simulink model "MPS_device_passive"  (R2018b)
settings: Solver=ode4  StartTime=0  StopTime=700  FixedStep=0.02  MaxStep=0.02  RelTol=1e-3  EnableMultiTasking=on
InitFcn:
  | %SSModel_calc
undefined symbols (not defined in the file): body, CentralPTOPreload, constraint, L, ML1Preload, ML2Preload, ML3Preload, ML4Preload, ML5Preload, ML6Preload, ML7Preload, ML8Preload, mrelative, pto, PTOrotation, SidePTO1Preload, SidePTO2Preload, SidePTO3Preload, SidePTO4Preload, simu, waves, X, Y, Z
libraries: nesl_utility x580, sm_lib x317, vrlib x72, WECSim_Lib x36
(part 26 of 27)

== matlab function MPS_device_passive/Control/Inverse Kinematic Jacobian - dynamic Go from 4 line forces to 6 Cartesian forces ==
  data: u input; y output
%Transform velocity or force from line space to cartesian space
%(underdetermined)

function y = dynamic_L(u)

rho_sea=1000;
g=9.81;
% Float
depth = 2;                  % Depth to top of float
Des = 12;                   % Outer diameter of float shell [m]
R = Des/2;                  % Outer radius of float shell [m]
CylLength = 4.75;           % Length of cylinder between hemispheres [m]
reldenfloat = 0.8;          % Density of float reative to sea water [-]
rho_steel = 7850;           % Density of steel [kg/m^3]
alphaDeg = 45;               % deg xz-plane (zero if att point is on horizontal central line, 90 if on bottom og float)
betaDeg = 0;               % deg xy-plane (zero if x value of att point is max (corner of cylinder) 90 y is max (peak of hemisphere))
FloatCd = 0.5;
FloatCdVector = [FloatCd 100 FloatCd 200*FloatCd 0 200*FloatCd];% Drag coefficients in 6 degrees of freedom, 4 and 6 picked at random to reduce yaw movement

% Reactor
ReactorD = 4.3;
ReactorCylLength = 35.7;                        % Only cylinder (excluding the two hemispheres)
ReactorWidth = 30;                              % From centre of tube to centre of tube
NetBuoyReactor = 101.9*10^3;                    % Net buoyancy of reactor [f kg] (Positive is buoyant)
ReactorDepth = 25.85;                           % Distance from mean sea surface to top of reactor (positive nr)
SeaDepth = 75;                                  % Distance from mean sea surface to seabed (positive nr)
ReactorCd = 0.5;
ReactorCdVector = [ReactorCd 100 ReactorCd 200*ReactorCd 200*ReactorCd 200*ReactorCd];   % Drag coefficients in 6 degrees of freedom, 4 and 6 picked at random to reduce yaw movement

%% Coordinates  (m, m, m)
% Tether line attachemnt point on float in global frame
%Transform to Float local frame - subtract float radius from z co-ord
%(Global frame at sea level)
F1 = [u(1) u(2) u(3)+8];
F2 = [u(4) u(5) u(6)+8];     % Corner tether
F3 = [u(7) u(8) u(9)+8];    % Corner tether
F4 = [u(10) u(11) u(12)+8];     % Corner tether

% Tether line attachemnt point on reactor in global frame
T1 = [ReactorCylLength/2 ReactorWidth/2 -ReactorDepth+depth+R];      % Corner tether transformed to relative to float COG
T2 = [T1(1) -T1(2) T1(3)];               % Corner tether
T3 = [-T1(1) -T1(2) T1(3)];              % Corner tether
T4 = [-T1(1) T1(2) T1(3)];               % Corner tether

%Vectors to float thether attachment points relative to float COG
N_01=[0 F1(3) -F1(2);-F1(3) 0 F1(1);F1(2) -F1(1) 0];
N_02=[0 F2(3) -F2(2);-F2(3) 0 F2(1);F2(2) -F2(1) 0];
N_03=[0 F3(3) -F3(2);-F3(3) 0 F3(1);F3(2) -F3(1) 0];
N_04=[0 F4(3) -F4(2);-F4(3) 0 F4(1);F4(2) -F4(1) 0];

%Vectors along PTO tethers
S1=F1-T1;
S2=F2-T2;
S3=F3-T3;
S4=F4-T4;

S_01=[0 S1(3) -S1(2);-S1(3) 0 S1(1);S1(2) -S1(1) 0];
S_02=[0 S2(3) -S2(2);-S2(3) 0 S2(1);S2(2) -S2(1) 0];
S_03=[0 S3(3) -S3(2);-S3(3) 0 S3(1);S3(2) -S3(1) 0];
S_04=[0 S4(3) -S4(2);-S4(3) 0 S4(1);S4(2) -S4(1) 0];

%Unit vectors along PTO tethers
e_s1=S1./norm(S1);
e_s2=S2./norm(S2);
e_s3=S3./norm(S3);
e_s4=S4./norm(S4);


%%%%Kt for non colinear lines
G_01 = -[eye(3);N_01']*e_s1';
G_02 = -[eye(3);N_02']*e_s2';
G_03 = -[eye(3);N_03']*e_s3';
G_04 = -[eye(3);N_04']*e_s4';

%Inverse kinematic Jacobian
L = -[G_01 G_02 G_03 G_04]';
y = L';

== matlab function MPS_device_passive/PTO P1F1/VisuP1F2/Hydrodynamic Body/Nonlinear Wave Elevation/Linear or Instantaneous Free Surface/Instantaneous Water Free Surface  /Instantaneous FS ==
  data: x input; center input; f output; cg input; AH input; w input; dw input; k input; typeNum input; t input; rampT input; phaseRand input; waveDir input; dt input; dtFe input
function f  = waveElevation(x,center,cg,AH,w,dw,k,typeNum,t,rampT,phaseRand,waveDir, dt, dtFe)
    % Function to calculate the wave elevation at the ceontroids of triangulated surface
    % NOTE: This function assumes that the STL file is imported with its CG at 0,0,0
    persistent oldElev
    if isempty(oldElev)
        f = calc_elev(x,center,cg,AH,w,dw,k,typeNum,t,rampT,phaseRand, waveDir);
        oldElev = f;
    else
        if mod(t, dtFe) < dt/2
            f = calc_elev(x,center,cg,AH,w,dw,k,typeNum,t,rampT,phaseRand, waveDir);
            oldElev = f;
        else
            f = oldElev;
        end
    end
end

function f = calc_elev(x,center,cg,AH,w,dw,k,typeNum,t,rampT,phaseRand,waveDir)
    % Function to rotate and translate body and call wave elevation function at new locations 
    
    % Compute new tri center coords after cog rotation and translation
    center = rotateXYZ(center,[1 0 0],x(4));
    center = rotateXYZ(center,[0 1 0],x(5));
    center = rotateXYZ(center,[0 0 1],x(6));
    center = offsetXYZ(center,x);
    center = offsetXYZ(center,cg);
    % Calculate the free surface
    f=waveElev(center,AH,w,dw,t,k,rampT,phaseRand,typeNum,waveDir);
end

function verts = offsetXYZ(verts,x)
    % Function to move the position vertices
    verts(:,1) = verts(:,1) + x(1);
    verts(:,2) = verts(:,2) + x(2);
    verts(:,3) = verts(:,3) + x(3);
end

function xn = rotateXYZ(x,ax,t)
	% Function to rotate a point about an arbitrary axis
	% x: 3-component coordinates
	% ax: axis about which to rotate (must be a vector length 1)
	% t: rotation angle
	% xn: new coordinates after rotation
	rotMat = zeros(3);
	rotMat(1,1) = ax(1)*ax(1)*(1-cos(t))    + cos(t);
	rotMat(1,2) = ax(2)*ax(1)*(1-cos(t))    + ax(3)*sin(t);
	rotMat(1,3) = ax(3)*ax(1)*(1-cos(t))    - ax(2)*sin(t);
	rotMat(2,1) = ax(1)*ax(2)*(1-cos(t))    - ax(3)*sin(t);
	rotMat(2,2) = ax(2)*ax(2)*(1-cos(t))    + cos(t);
	rotMat(2,3) = ax(3)*ax(2)*(1-cos(t))    + ax(1)*sin(t);
	rotMat(3,1) = ax(1)*ax(3)*(1-cos(t))    + ax(2)*sin(t);
	rotMat(3,2) = ax(2)*ax(3)*(1-cos(t))    - ax(1)*sin(t);
	rotMat(3,3) = ax(3)*ax(3)*(1-cos(t))    + cos(t);
	xn = x*rotMat;
end

function f=waveElev(center,AH,w,dw,t,k,rampT,phaseRand,typeNum,waveDir)
    % Function to calculate the wave elevation at an array of points
    f = zeros(length(center(:,3)),1);
    cx = center(:,1);
    cy = center(:,2);
    X = cx*cos(waveDir*pi/180) + cy*sin(waveDir*pi/180);
    if typeNum <10
    elseif typeNum <20
        f = AH(1).*cos(k(1).*X-w(1)*t);
    elseif typeNum <30
        tmp=sqrt(AH.*dw);
        tmp1 = ones(1,length(center(:,1)));
        tmp2 = (w.*t+phaseRand)*tmp1;
        tmp3 = cos(k*X'- tmp2);
        f(:,1) = tmp3'*tmp;
    end
    if t<=rampT
        rampF = (1+cos(pi+pi*t/rampT))/2;
        f = f.*rampF;
    end
end

== matlab function MPS_device_passive/PTO P1F1/VisuP1F2/Hydrodynamic Body/Structure/Motion Sensor/Angle ==
  data: Q input; E output
function E  = EulerAngle(Q)
% Euler Angle Type II or Tait-Bryan Angle for sequence 321 or zyx (Nautical or Cardan angles).
% Yaw [-180,180], followed by pitch [-90,90], followed by roll [-180,180]
E = zeros(3,1);
E(1) = atan2((2*(Q(1)*Q(2)+Q(3)*Q(4))),(1-2*(Q(2)^2+Q(3)^2)));
E(2) = asin(2*(Q(1)*Q(3)-Q(4)*Q(2)));
E(3) = atan2((2*(Q(1)*Q(4)+Q(2)*Q(3))),(1-2*(Q(3)^2+Q(4)^2)));

== matlab function MPS_device_passive/PTO P1F1/VisuP1F2/Hydrodynamic Body/Wave Diffraction and Excitation Force Calculation/Linear Wave Excitation Force Variant Subsystem/Irregular Wave Excitation Force/MATLAB Function ==
  data: A input; Fext output; w input; fExtRE input; fExtIM input; phaseRand input; dw input; time input
function Fext = fcn(A,w,fExtRE,fExtIM,phaseRand,dw,time)
%#codegen

persistent A1 B1 B11 C1 D1 D11 E1 E11

A1=bsxfun(@plus,w*time,pi/2);
B1= sin(bsxfun(@plus,A1,phaseRand));
B11 = sin(bsxfun(@plus,w*time,phaseRand));
C1 = sqrt(bsxfun(@times,A,dw));
D1 =bsxfun(@times,fExtRE,C1);
D11 = bsxfun(@times,fExtIM,C1);
E1 = bsxfun(@times,B1,D1);
E11 = bsxfun(@times,B11,D11);

Fext = sum(bsxfun(@minus,E1,E11));

== matlab function MPS_device_passive/PTO P1F1/VisuP1F2/Hydrodynamic Body/Wave Diffraction and Excitation Force Calculation/Nonlinear FK Force Variant Subsystem/With Nonlinear FroudeKrylov Force/Diffraction and Excitation Forces ==
  data: x input; elv input; center input; f output; tnorm input; area input; rho input; g input; cg input; AH input; w input; dw input; wDepth input; deepWaterWave input; k input; typeNum input; t input; phaseRand input; wp output; wpMeanFS output; dt input; dtFe input
function [f, wp, wpMeanFS]  = nonFKForce(x,elv,center,tnorm,area,rho,g,cg,AH,w,dw,wDepth,deepWaterWave,k,typeNum,t,phaseRand, dt, dtFe)
    % Function to calculate wave exitation force and moment on a triangulated surface
    % NOTE: This function assumes that the STL file is imported with its CG at 0,0,0
    
    % Logic to calculate nonFKForce at reduced sample time
    persistent oldForce
    persistent oldWp
    persistent oldWpMeanFs
    
    if isempty(oldForce)
        [f, wp, wpMeanFS] = calc_force(x,elv,center,tnorm,area,rho,g,cg,AH,w,dw,wDepth,deepWaterWave,k,typeNum,t,phaseRand);
        oldForce = f;
        oldWp = wp;
        oldWpMeanFs = wpMeanFS;
    else
        if mod(t, dtFe) < dt/2
            [f, wp, wpMeanFS] = calc_force(x,elv,center,tnorm,area,rho,g,cg,AH,w,dw,wDepth,deepWaterWave,k,typeNum,t,phaseRand);
            oldForce = f;
            oldWp = wp;
            oldWpMeanFs = wpMeanFS;
        else
            f = oldForce;
            wp = oldWp;
            wpMeanFS = oldWpMeanFs;
        end
    end
end

function [f, wp, wpMeanFS]  = calc_force(x,elv,center,tnorm,area,rho,g,cg,AH,w,dw,wDepth,deepWaterWave,k,typeNum,t,phaseRand)
    % Function to apply translation and rotation, and calculate forces.
    
    % Compute new tri coords after cog rotation and translation
    centerMeanFS = offsetXYZ(center,cg);
    avMeanFS     = tnorm .* [area area area];
    
    % Compute new tri coords after cog rotation and translation
    center = rotateXYZ(center,[1 0 0],x(4));
    center = rotateXYZ(center,[0 1 0],x(5));
    center = rotateXYZ(center,[0 0 1],x(6));
    center = offsetXYZ(center,x);
    center = offsetXYZ(center,cg);
    % Compute new normal vectors coords after cog rotation and translation
    tnorm = rotateXYZ(tnorm,[1 0 0],x(4));
    tnorm = rotateXYZ(tnorm,[0 1 0],x(5));
    tnorm = rotateXYZ(tnorm,[0 0 1],x(6));
    
    % Copute area vectors
    av = tnorm .* [area area area];
    
    % Calculate the free surface
    wpMeanFS=pDis(centerMeanFS,       0,AH,w,dw,wDepth,deepWaterWave,t,k,phaseRand,typeNum,rho,g);
    wp      =pDis(center      ,     elv,AH,w,dw,wDepth,deepWaterWave,t,k,phaseRand,typeNum,rho,g);
    
    % Calculate forces
    f_linear   =FK(centerMeanFS,       cg,avMeanFS,wpMeanFS);
    f_nonLinear=FK(center      ,x(1:3)+cg,av      ,wp      ); 
    f = f_nonLinear-f_linear;
end

function verts = offsetXYZ(verts,x)
    % Function to move the position vertices
    verts(:,1) = verts(:,1) + x(1);
    verts(:,2) = verts(:,2) + x(2);
    verts(:,3) = verts(:,3) + x(3);
end

function xn = rotateXYZ(x,ax,t)
	% Function to rotate a point about an arbitrary axis
	% x: 3-componenet coordinates
	% ax: axis about which to rotate (must be a vector length 1)
	% t: rotation angle
	% xn: new coordinates after rotation
	rotMat = zeros(3);
	rotMat(1,1) = ax(1)*ax(1)*(1-cos(t))    + cos(t);
	rotMat(1,2) = ax(2)*ax(1)*(1-cos(t))    + ax(3)*sin(t);
	rotMat(1,3) = ax(3)*ax(1)*(1-cos(t))    - ax(2)*sin(t);
	rotMat(2,1) = ax(1)*ax(2)*(1-cos(t))    - ax(3)*sin(t);
	rotMat(2,2) = ax(2)*ax(2)*(1-cos(t))    + cos(t);
	rotMat(2,3) = ax(3)*ax(2)*(1-cos(t))    + ax(1)*sin(t);
	rotMat(3,1) = ax(1)*ax(3)*(1-cos(t))    + ax(2)*sin(t);
	rotMat(3,2) = ax(2)*ax(3)*(1-cos(t))    - ax(1)*sin(t);
	rotMat(3,3) = ax(3)*ax(3)*(1-cos(t))    + cos(t);
	xn = x*rotMat;
end

function f=pDis(center,elv,AH,w,dw,wDepth,deepWaterWave,t,k,phaseRand,typeNum,rho,g)
    % Function to calculate pressure distribution
    f = zeros(length(center(:,3)),1);
    z=zeros(length(center(:,1)),1);
    if typeNum <10
    elseif typeNum <20
        f = rho.*g.*AH(1).*cos(k(1).*center(:,1)-w(1)*t);
        if deepWaterWave == 0
            z=(center(:,3)-elv).*wDepth./(wDepth+elv);
            f = f.*(cosh(k(1).*(z+wDepth))./cosh(k(1)*wDepth));
        else
            z=(center(:,3)-elv);
            f = f.*exp(k(1).*z);
        end
    elseif typeNum <30
        for i=1:length(AH)
            if deepWaterWave == 0 && wDepth <= 0.5*pi/k(i)
                z=(center(:,3)-elv).*wDepth./(wDepth+elv);
                f_tmp = rho.*g.*sqrt(AH(i)*dw).*cos(k(i).*center(:,1)-w(i)*t-phaseRand(i));
                f = f + f_tmp.*(cosh(k(i).*(z+wDepth))./cosh(k(i).*wDepth));
            else
                z=(center(:,3)-elv);
                f_tmp = rho.*g.*sqrt(AH(i)*dw).*cos(k(i).*center(:,1)-w(i)*t-phaseRand(i));
                f = f + f_tmp.*exp(k(i).*z);
            end
        end
    end
    f(z>0)=0;
end

function f = FK(center,instcg,av,wp)
    % Function to calculate the force and moment about the cog due to Froude-Krylov pressure
    f = zeros(6,1);
    
    % Calculate the hydrostatic pressure at each triangle center
    pressureVect = [wp wp wp].*-av;
    
    % Compute force about cog
    f(1:3) = sum(pressureVect);
    
    % Compute moment about cog
    tmp1 = ones(length(center(:,1)),1);
    tmp2 = tmp1*instcg';
    center2cgVec = center-tmp2;
    
    f(4:6)= sum(cross(center2cgVec,pressureVect));
end

== matlab function MPS_device_passive/PTO P1F1/VisuP1F2/Hydrodynamic Body/Wave Radiation Forces Calculation/SS CI and Constant-Damping-CoeVariant Subsystem/Convolution Integral Calculation/Fluid Memory ==
  data: lenJ input; v input; F_FM output; IRKB input; CTTime input; clockTime input
function F_FM = ConvolutionIntegral(lenJ,v,IRKB,CTTime,clockTime)
% Function to calculate convolution integral
interp_factor = 1;
%define persistent variables
persistent velocity;
persistent oldTime;
persistent oldF_FM;
persistent IRKB_interp;

dt = CTTime(2)-CTTime(1);
len = length(CTTime);
lenJ=length(lenJ);

%update velocity
if isempty(velocity)
    velocity = zeros(lenJ,len);
    oldTime = 0;
    F_FM    = zeros(6,1);
    oldF_FM = zeros(6,1);
    IRKB_reordered = permute(IRKB,[3 1 2]);
    IRKB_interp    = IRKB_reordered(:,1:interp_factor:end, :);
else
    if abs(clockTime-oldTime-dt)<0.00000001
        velocity      = circshift(velocity, 1, 2);
        velocity(:,1) = v(:);
        %integrate       
        time_series = bsxfun(@times, IRKB_interp, velocity);
        F_FM =squeeze(trapz(CTTime,sum(time_series, 1)));
         oldF_FM = F_FM;
         oldTime = clockTime;
    else
        F_FM = oldF_FM;
    end
end

end

== matlab function MPS_device_passive/PTO P1F1/VisuP1F2/Non-Hydro Body/Structure/Motion Sensor/Angle ==
  data: Q input; E output
function E  = EulerAngle(Q)
% Euler Angle Type II or Tait-Bryan Angle for sequence 321 or zyx (Nautical or Cardan angles).
% Yaw [-180,180], followed by pitch [-90,90], followed by roll [-180,180]
E = zeros(3,1);
E(1) = atan2( (2*(Q(1)*Q(2)+Q(3)*Q(4))), (1-2* (Q(2)^2+Q(3)^2) ) );
E(2) = asin( 2* (Q(1)*Q(3) - Q(4)*Q(2)));
E(3) = atan2( (2*(Q(1)*Q(4)+Q(2)*Q(3))), (1-2* (Q(3)^2+Q(4)^2) ) );

== matlab function MPS_device_passive/PTO P2F2/VisuP2F3/Hydrodynamic Body/Hydrostatic Restoring Force Calculation/Linear and Nonlinear Restoring Force Variant Subsystem/Nonlinear Hydrostatic Restoring Force/Diffarction and Excitation Forces1 ==
  data: x input; elv input; center input; f output; tnorm input; area input; rho input; g input; cg input; p output; dt input; dtFe input; t input
function [f,p]  = nonLinearBuoyancy(x,elv,center,tnorm,area,rho,g,cg,dt,dtFe,t)
% Function to calculate buoyancy force and moment on a triangulated surface
% NOTE: This function assumes that the STL file is imported with its CG at 0,0,0
persistent oldF 
persistent oldP

if isempty(oldF)
    [f,p] = calc_buoyancy(x,elv,center,tnorm,area,rho,g,cg);
    oldF  = f;
    oldP  = p;
else
    if mod(t, dtFe) < dt/2
        [f,p] = calc_buoyancy(x,elv,center,tnorm,area,rho,g,cg);
        oldF  = f;
        oldP  = p;
    else
        f  = oldF;
        p  = oldP;
    end
end
end


function [f,p] = calc_buoyancy(x,elv,center,tnorm,area,rho,g,cg)
% Function to apply translation and rotation and calculate forces

% Compute new tri coords after cog rotation and translation
center = rotateXYZ(center,[1 0 0],x(4));
center = rotateXYZ(center,[0 1 0],x(5));
center = rotateXYZ(center,[0 0 1],x(6));
center = offsetXYZ(center,x);
center = offsetXYZ(center,cg);
% Compute new normal vectors coords after cog rotation
tnorm = rotateXYZ(tnorm,[1 0 0],x(4));
tnorm = rotateXYZ(tnorm,[0 1 0],x(5));
tnorm = rotateXYZ(tnorm,[0 0 1],x(6));

% Calculate the hydrostatic forces
av = tnorm .* [area area area];
[f,p]=fHydrostatic(center,elv,x(1:3)+cg,av,rho,g); 
end

function verts = offsetXYZ(verts,x)
% Function to move the position vertices
verts(:,1) = verts(:,1) + x(1);
verts(:,2) = verts(:,2) + x(2);
verts(:,3) = verts(:,3) + x(3);
end

function xn = rotateXYZ(x,ax,t)
	% Function to rotate a point about an arbitrary axis
	% x: 3-componenet coordiantes
	% ax: axis about which to rotate (must be a vector length 1)
	% t: rotation angle
	% xn: new coordinates after rotation
	rotMat = zeros(3);
	rotMat(1,1) = ax(1)*ax(1)*(1-cos(t))    + cos(t);
	rotMat(1,2) = ax(2)*ax(1)*(1-cos(t))    + ax(3)*sin(t);
	rotMat(1,3) = ax(3)*ax(1)*(1-cos(t))    - ax(2)*sin(t);
	rotMat(2,1) = ax(1)*ax(2)*(1-cos(t))    - ax(3)*sin(t);
	rotMat(2,2) = ax(2)*ax(2)*(1-cos(t))    + cos(t);
	rotMat(2,3) = ax(3)*ax(2)*(1-cos(t))    + ax(1)*sin(t);
	rotMat(3,1) = ax(1)*ax(3)*(1-cos(t))    + ax(2)*sin(t);
	rotMat(3,2) = ax(2)*ax(3)*(1-cos(t))    - ax(1)*sin(t);
	rotMat(3,3) = ax(3)*ax(3)*(1-cos(t))    + cos(t);
	xn = x*rotMat;
end

function [f,p] = fHydrostatic(center,elv,instcg,av,rho,g)
% Function to calculate the force and moment about the cog due to hydrostatic pressure
f = zeros(6,1);

% Zeor out regions above the mean free surface
z=center(:,3); z((z-elv)>0)=0;

% Calculate the hydrostatic pressure at each triangle center
pressureVect = rho*g.*[-z -z -z].*-av;
p = rho*g.*-z;
% Compute force about cog
f(1:3) = sum(pressureVect);

tmp1 = ones(length(center(:,1)),1);
tmp2 = tmp1*instcg';
center2cgVec = center-tmp2;

f(4:6)= sum(cross(center2cgVec,pressureVect));
end

== matlab function MPS_device_passive/PTO P2F2/VisuP2F3/Hydrodynamic Body/Morrison Element and ViscousDampingForceCalculation/Morrison Element Variant Subsystem/Morrison Element On/Irregular Wave Morison Force/MorrisonElements/MorisonElementIrregular/MATLAB Function ==
  data: u output; v output; disp input size=[1 3]; waveNumber input; waveFreq input; waveAmp input; randPhase input; time input; rampT input size=[1 1]; waveDir input size=[1 1]; waterDepth input size=[1 1]; g input size=[1 1]; w output; xa output; ya output; za output
function [u,v,w,xa,ya,za] = calc_orbital_vel(disp, waveNumber, waveFreq, waveAmp, randPhase, time, rampT, waveDir, waterDepth, g)
%#codegen

[u,v,w,xa,ya,za] = orbital_velocity(disp, waveNumber, waveFreq, waveAmp, randPhase, time, rampT, waveDir, waterDepth, g);

== matlab function MPS_device_passive/PTO P2F2/VisuP2F3/Hydrodynamic Body/Morrison Element and ViscousDampingForceCalculation/Morrison Element Variant Subsystem/Morrison Element On/Regular Wave Morison Force/MorrisonElements/OrbitalVelocity/MATLAB Function ==
  data: u output; v output; disp input size=[1 3]; waveNumber input size=[1 1]; waveFreq input size=[1 1]; waveAmp input size=[1 1]; randPhase input; time input; rampT input size=[1 1]; waveDir input size=[1 1]; waterDepth input size=[1 1]; g input size=[1 1]; w output; xa output; ya output; za output
function [u,v,w,xa,ya,za] = calc_orbital_vel(disp, waveNumber, waveFreq, waveAmp, randPhase, time, rampT, waveDir, waterDepth, g)
%#codegen

[u,v,w,xa,ya,za] = orbital_velocity(disp, waveNumber, waveFreq, waveAmp, randPhase, time, rampT, waveDir, waterDepth, g);

== matlab function MPS_device_passive/PTO P2F2/VisuP2F3/Hydrodynamic Body/Nonlinear Wave Elevation/Linear or Instantaneous Free Surface/Instantaneous Water Free Surface  /Instantaneous FS ==
  data: x input; center input; f output; cg input; AH input; w input; dw input; k input; typeNum input; t input; rampT input; phaseRand input; waveDir input; dt input; dtFe input
function f  = waveElevation(x,center,cg,AH,w,dw,k,typeNum,t,rampT,phaseRand,waveDir, dt, dtFe)
    % Function to calculate the wave elevation at the ceontroids of triangulated surface
    % NOTE: This function assumes that the STL file is imported with its CG at 0,0,0
    persistent oldElev
    if isempty(oldElev)
        f = calc_elev(x,center,cg,AH,w,dw,k,typeNum,t,rampT,phaseRand, waveDir);
        oldElev = f;
    else
        if mod(t, dtFe) < dt/2
            f = calc_elev(x,center,cg,AH,w,dw,k,typeNum,t,rampT,phaseRand, waveDir);
            oldElev = f;
        else
            f = oldElev;
        end
    end
end

function f = calc_elev(x,center,cg,AH,w,dw,k,typeNum,t,rampT,phaseRand,waveDir)
    % Function to rotate and translate body and call wave elevation function at new locations 
    
    % Compute new tri center coords after cog rotation and translation
    center = rotateXYZ(center,[1 0 0],x(4));
    center = rotateXYZ(center,[0 1 0],x(5));
    center = rotateXYZ(center,[0 0 1],x(6));
    center = offsetXYZ(center,x);
    center = offsetXYZ(center,cg);
    % Calculate the free surface
    f=waveElev(center,AH,w,dw,t,k,rampT,phaseRand,typeNum,waveDir);
end

function verts = offsetXYZ(verts,x)
    % Function to move the position vertices
    verts(:,1) = verts(:,1) + x(1);
    verts(:,2) = verts(:,2) + x(2);
    verts(:,3) = verts(:,3) + x(3);
end

function xn = rotateXYZ(x,ax,t)
	% Function to rotate a point about an arbitrary axis
	% x: 3-component coordinates
	% ax: axis about which to rotate (must be a vector length 1)
	% t: rotation angle
	% xn: new coordinates after rotation
	rotMat = zeros(3);
	rotMat(1,1) = ax(1)*ax(1)*(1-cos(t))    + cos(t);
	rotMat(1,2) = ax(2)*ax(1)*(1-cos(t))    + ax(3)*sin(t);
	rotMat(1,3) = ax(3)*ax(1)*(1-cos(t))    - ax(2)*sin(t);
	rotMat(2,1) = ax(1)*ax(2)*(1-cos(t))    - ax(3)*sin(t);
	rotMat(2,2) = ax(2)*ax(2)*(1-cos(t))    + cos(t);
	rotMat(2,3) = ax(3)*ax(2)*(1-cos(t))    + ax(1)*sin(t);
	rotMat(3,1) = ax(1)*ax(3)*(1-cos(t))    + ax(2)*sin(t);
	rotMat(3,2) = ax(2)*ax(3)*(1-cos(t))    - ax(1)*sin(t);
	rotMat(3,3) = ax(3)*ax(3)*(1-cos(t))    + cos(t);
	xn = x*rotMat;
end

function f=waveElev(center,AH,w,dw,t,k,rampT,phaseRand,typeNum,waveDir)
    % Function to calculate the wave elevation at an array of points
    f = zeros(length(center(:,3)),1);
    cx = center(:,1);
    cy = center(:,2);
    X = cx*cos(waveDir*pi/180) + cy*sin(waveDir*pi/180);
    if typeNum <10
    elseif typeNum <20
        f = AH(1).*cos(k(1).*X-w(1)*t);
    elseif typeNum <30
        tmp=sqrt(AH.*dw);
        tmp1 = ones(1,length(center(:,1)));
        tmp2 = (w.*t+phaseRand)*tmp1;
        tmp3 = cos(k*X'- tmp2);
        f(:,1) = tmp3'*tmp;
    end
    if t<=rampT
        rampF = (1+cos(pi+pi*t/rampT))/2;
        f = f.*rampF;
    end
end

== matlab function MPS_device_passive/PTO P2F2/VisuP2F3/Hydrodynamic Body/Structure/Motion Sensor/Angle ==
  data: Q input; E output
function E  = EulerAngle(Q)
% Euler Angle Type II or Tait-Bryan Angle for sequence 321 or zyx (Nautical or Cardan angles).
% Yaw [-180,180], followed by pitch [-90,90], followed by roll [-180,180]
E = zeros(3,1);
E(1) = atan2((2*(Q(1)*Q(2)+Q(3)*Q(4))),(1-2*(Q(2)^2+Q(3)^2)));
E(2) = asin(2*(Q(1)*Q(3)-Q(4)*Q(2)));
E(3) = atan2((2*(Q(1)*Q(4)+Q(2)*Q(3))),(1-2*(Q(3)^2+Q(4)^2)));

== matlab function MPS_device_passive/PTO P2F2/VisuP2F3/Hydrodynamic Body/Wave Diffraction and Excitation Force Calculation/Linear Wave Excitation Force Variant Subsystem/Irregular Wave Excitation Force/MATLAB Function ==
  data: A input; Fext output; w input; fExtRE input; fExtIM input; phaseRand input; dw input; time input
function Fext = fcn(A,w,fExtRE,fExtIM,phaseRand,dw,time)
%#codegen

persistent A1 B1 B11 C1 D1 D11 E1 E11

A1=bsxfun(@plus,w*time,pi/2);
B1= sin(bsxfun(@plus,A1,phaseRand));
B11 = sin(bsxfun(@plus,w*time,phaseRand));
C1 = sqrt(bsxfun(@times,A,dw));
D1 =bsxfun(@times,fExtRE,C1);
D11 = bsxfun(@times,fExtIM,C1);
E1 = bsxfun(@times,B1,D1);
E11 = bsxfun(@times,B11,D11);

Fext = sum(bsxfun(@minus,E1,E11));

== matlab function MPS_device_passive/PTO P2F2/VisuP2F3/Hydrodynamic Body/Wave Diffraction and Excitation Force Calculation/Nonlinear FK Force Variant Subsystem/With Nonlinear FroudeKrylov Force/Diffraction and Excitation Forces ==
  data: x input; elv input; center input; f output; tnorm input; area input; rho input; g input; cg input; AH input; w input; dw input; wDepth input; deepWaterWave input; k input; typeNum input; t input; phaseRand input; wp output; wpMeanFS output; dt input; dtFe input
function [f, wp, wpMeanFS]  = nonFKForce(x,elv,center,tnorm,area,rho,g,cg,AH,w,dw,wDepth,deepWaterWave,k,typeNum,t,phaseRand, dt, dtFe)
    % Function to calculate wave exitation force and moment on a triangulated surface
    % NOTE: This function assumes that the STL file is imported with its CG at 0,0,0
    
    % Logic to calculate nonFKForce at reduced sample time
    persistent oldForce
    persistent oldWp
    persistent oldWpMeanFs
    
    if isempty(oldForce)
        [f, wp, wpMeanFS] = calc_force(x,elv,center,tnorm,area,rho,g,cg,AH,w,dw,wDepth,deepWaterWave,k,typeNum,t,phaseRand);
        oldForce = f;
        oldWp = wp;
        oldWpMeanFs = wpMeanFS;
    else
        if mod(t, dtFe) < dt/2
            [f, wp, wpMeanFS] = calc_force(x,elv,center,tnorm,area,rho,g,cg,AH,w,dw,wDepth,deepWaterWave,k,typeNum,t,phaseRand);
            oldForce = f;
            oldWp = wp;
            oldWpMeanFs = wpMeanFS;
        else
            f = oldForce;
            wp = oldWp;
            wpMeanFS = oldWpMeanFs;
        end
    end
end

function [f, wp, wpMeanFS]  = calc_force(x,elv,center,tnorm,area,rho,g,cg,AH,w,dw,wDepth,deepWaterWave,k,typeNum,t,phaseRand)
    % Function to apply translation and rotation, and calculate forces.
    
    % Compute new tri coords after cog rotation and translation
    centerMeanFS = offsetXYZ(center,cg);
    avMeanFS     = tnorm .* [area area area];
    
    % Compute new tri coords after cog rotation and translation
    center = rotateXYZ(center,[1 0 0],x(4));
    center = rotateXYZ(center,[0 1 0],x(5));
    center = rotateXYZ(center,[0 0 1],x(6));
    center = offsetXYZ(center,x);
    center = offsetXYZ(center,cg);
    % Compute new normal vectors coords after cog rotation and translation
    tnorm = rotateXYZ(tnorm,[1 0 0],x(4));
    tnorm = rotateXYZ(tnorm,[0 1 0],x(5));
    tnorm = rotateXYZ(tnorm,[0 0 1],x(6));
    
    % Copute area vectors
    av = tnorm .* [area area area];
    
    % Calculate the free surface
    wpMeanFS=pDis(centerMeanFS,       0,AH,w,dw,wDepth,deepWaterWave,t,k,phaseRand,typeNum,rho,g);
    wp      =pDis(center      ,     elv,AH,w,dw,wDepth,deepWaterWave,t,k,phaseRand,typeNum,rho,g);
    
    % Calculate forces
    f_linear   =FK(centerMeanFS,       cg,avMeanFS,wpMeanFS);
    f_nonLinear=FK(center      ,x(1:3)+cg,av      ,wp      ); 
    f = f_nonLinear-f_linear;
end

function verts = offsetXYZ(verts,x)
    % Function to move the position vertices
    verts(:,1) = verts(:,1) + x(1);
    verts(:,2) = verts(:,2) + x(2);
    verts(:,3) = verts(:,3) + x(3);
end

function xn = rotateXYZ(x,ax,t)
	% Function to rotate a point about an arbitrary axis
	% x: 3-componenet coordinates
	% ax: axis about which to rotate (must be a vector length 1)
	% t: rotation angle
	% xn: new coordinates after rotation
	rotMat = zeros(3);
	rotMat(1,1) = ax(1)*ax(1)*(1-cos(t))    + cos(t);
	rotMat(1,2) = ax(2)*ax(1)*(1-cos(t))    + ax(3)*sin(t);
	rotMat(1,3) = ax(3)*ax(1)*(1-cos(t))    - ax(2)*sin(t);
	rotMat(2,1) = ax(1)*ax(2)*(1-cos(t))    - ax(3)*sin(t);
	rotMat(2,2) = ax(2)*ax(2)*(1-cos(t))    + cos(t);
	rotMat(2,3) = ax(3)*ax(2)*(1-cos(t))    + ax(1)*sin(t);
	rotMat(3,1) = ax(1)*ax(3)*(1-cos(t))    + ax(2)*sin(t);
	rotMat(3,2) = ax(2)*ax(3)*(1-cos(t))    - ax(1)*sin(t);
	rotMat(3,3) = ax(3)*ax(3)*(1-cos(t))    + cos(t);
	xn = x*rotMat;
end

function f=pDis(center,elv,AH,w,dw,wDepth,deepWaterWave,t,k,phaseRand,typeNum,rho,g)
    % Function to calculate pressure distribution
    f = zeros(length(center(:,3)),1);
    z=zeros(length(center(:,1)),1);
    if typeNum <10
    elseif typeNum <20
        f = rho.*g.*AH(1).*cos(k(1).*center(:,1)-w(1)*t);
        if deepWaterWave == 0
            z=(center(:,3)-elv).*wDepth./(wDepth+elv);
            f = f.*(cosh(k(1).*(z+wDepth))./cosh(k(1)*wDepth));
        else
            z=(center(:,3)-elv);
            f = f.*exp(k(1).*z);
        end
    elseif typeNum <30
        for i=1:length(AH)
            if deepWaterWave == 0 && wDepth <= 0.5*pi/k(i)
                z=(center(:,3)-elv).*wDepth./(wDepth+elv);
                f_tmp = rho.*g.*sqrt(AH(i)*dw).*cos(k(i).*center(:,1)-w(i)*t-phaseRand(i));
                f = f + f_tmp.*(cosh(k(i).*(z+wDepth))./cosh(k(i).*wDepth));
            else
                z=(center(:,3)-elv);
                f_tmp = rho.*g.*sqrt(AH(i)*dw).*cos(k(i).*center(:,1)-w(i)*t-phaseRand(i));
                f = f + f_tmp.*exp(k(i).*z);
            end
        end
    end
    f(z>0)=0;
end

function f = FK(center,instcg,av,wp)
    % Function to calculate the force and moment about the cog due to Froude-Krylov pressure
    f = zeros(6,1);
    
    % Calculate the hydrostatic pressure at each triangle center
    pressureVect = [wp wp wp].*-av;
    
    % Compute force about cog
    f(1:3) = sum(pressureVect);
    
    % Compute moment about cog
    tmp1 = ones(length(center(:,1)),1);
    tmp2 = tmp1*instcg';
    center2cgVec = center-tmp2;
    
    f(4:6)= sum(cross(center2cgVec,pressureVect));
end

== matlab function MPS_device_passive/PTO P2F2/VisuP2F3/Hydrodynamic Body/Wave Radiation Forces Calculation/SS CI and Constant-Damping-CoeVariant Subsystem/Convolution Integral Calculation/Fluid Memory ==
  data: lenJ input; v input; F_FM output; IRKB input; CTTime input; clockTime input
function F_FM = ConvolutionIntegral(lenJ,v,IRKB,CTTime,clockTime)
% Function to calculate convolution integral
interp_factor = 1;
%define persistent variables
persistent velocity;
persistent oldTime;
persistent oldF_FM;
persistent IRKB_interp;

dt = CTTime(2)-CTTime(1);
len = length(CTTime);
lenJ=length(lenJ);

%update velocity
if isempty(velocity)
    velocity = zeros(lenJ,len);
    oldTime = 0;
    F_FM    = zeros(6,1);
    oldF_FM = zeros(6,1);
    IRKB_reordered = permute(IRKB,[3 1 2]);
    IRKB_interp    = IRKB_reordered(:,1:interp_factor:end, :);
else
    if abs(clockTime-oldTime-dt)<0.00000001
        velocity      = circshift(velocity, 1, 2);
        velocity(:,1) = v(:);
        %integrate       
        time_series = bsxfun(@times, IRKB_interp, velocity);
        F_FM =squeeze(trapz(CTTime,sum(time_series, 1)));
         oldF_FM = F_FM;
         oldTime = clockTime;
    else
        F_FM = oldF_FM;
    end
end

end

== matlab function MPS_device_passive/PTO P2F2/VisuP2F3/Non-Hydro Body/Structure/Motion Sensor/Angle ==
  data: Q input; E output
function E  = EulerAngle(Q)
% Euler Angle Type II or Tait-Bryan Angle for sequence 321 or zyx (Nautical or Cardan angles).
% Yaw [-180,180], followed by pitch [-90,90], followed by roll [-180,180]
E = zeros(3,1);
E(1) = atan2( (2*(Q(1)*Q(2)+Q(3)*Q(4))), (1-2* (Q(2)^2+Q(3)^2) ) );
E(2) = asin( 2* (Q(1)*Q(3) - Q(4)*Q(2)));
E(3) = atan2( (2*(Q(1)*Q(4)+Q(2)*Q(3))), (1-2* (Q(3)^2+Q(4)^2) ) );

== matlab function MPS_device_passive/PTO P3F3/VisuP3F2/Hydrodynamic Body/Hydrostatic Restoring Force Calculation/Linear and Nonlinear Restoring Force Variant Subsystem/Nonlinear Hydrostatic Restoring Force/Diffarction and Excitation Forces1 ==
  data: x input; elv input; center input; f output; tnorm input; area input; rho input; g input; cg input; p output; dt input; dtFe input; t input
function [f,p]  = nonLinearBuoyancy(x,elv,center,tnorm,area,rho,g,cg,dt,dtFe,t)
% Function to calculate buoyancy force and moment on a triangulated surface
% NOTE: This function assumes that the STL file is imported with its CG at 0,0,0
persistent oldF 
persistent oldP

if isempty(oldF)
    [f,p] = calc_buoyancy(x,elv,center,tnorm,area,rho,g,cg);
    oldF  = f;
    oldP  = p;
else
    if mod(t, dtFe) < dt/2
        [f,p] = calc_buoyancy(x,elv,center,tnorm,area,rho,g,cg);
        oldF  = f;
        oldP  = p;
    else
        f  = oldF;
        p  = oldP;
    end
end
end


function [f,p] = calc_buoyancy(x,elv,center,tnorm,area,rho,g,cg)
% Function to apply translation and rotation and calculate forces

% Compute new tri coords after cog rotation and translation
center = rotateXYZ(center,[1 0 0],x(4));
center = rotateXYZ(center,[0 1 0],x(5));
center = rotateXYZ(center,[0 0 1],x(6));
center = offsetXYZ(center,x);
center = offsetXYZ(center,cg);
% Compute new normal vectors coords after cog rotation
tnorm = rotateXYZ(tnorm,[1 0 0],x(4));
tnorm = rotateXYZ(tnorm,[0 1 0],x(5));
tnorm = rotateXYZ(tnorm,[0 0 1],x(6));

% Calculate the hydrostatic forces
av = tnorm .* [area area area];
[f,p]=fHydrostatic(center,elv,x(1:3)+cg,av,rho,g); 
end

function verts = offsetXYZ(verts,x)
% Function to move the position vertices
verts(:,1) = verts(:,1) + x(1);
verts(:,2) = verts(:,2) + x(2);
verts(:,3) = verts(:,3) + x(3);
end

function xn = rotateXYZ(x,ax,t)
	% Function to rotate a point about an arbitrary axis
	% x: 3-componenet coordiantes
	% ax: axis about which to rotate (must be a vector length 1)
	% t: rotation angle
	% xn: new coordinates after rotation
	rotMat = zeros(3);
	rotMat(1,1) = ax(1)*ax(1)*(1-cos(t))    + cos(t);
	rotMat(1,2) = ax(2)*ax(1)*(1-cos(t))    + ax(3)*sin(t);
	rotMat(1,3) = ax(3)*ax(1)*(1-cos(t))    - ax(2)*sin(t);
	rotMat(2,1) = ax(1)*ax(2)*(1-cos(t))    - ax(3)*sin(t);
	rotMat(2,2) = ax(2)*ax(2)*(1-cos(t))    + cos(t);
	rotMat(2,3) = ax(3)*ax(2)*(1-cos(t))    + ax(1)*sin(t);
	rotMat(3,1) = ax(1)*ax(3)*(1-cos(t))    + ax(2)*sin(t);
	rotMat(3,2) = ax(2)*ax(3)*(1-cos(t))    - ax(1)*sin(t);
	rotMat(3,3) = ax(3)*ax(3)*(1-cos(t))    + cos(t);
	xn = x*rotMat;
end

function [f,p] = fHydrostatic(center,elv,instcg,av,rho,g)
% Function to calculate the force and moment about the cog due to hydrostatic pressure
f = zeros(6,1);

% Zeor out regions above the mean free surface
z=center(:,3); z((z-elv)>0)=0;

% Calculate the hydrostatic pressure at each triangle center
pressureVect = rho*g.*[-z -z -z].*-av;
p = rho*g.*-z;
% Compute force about cog
f(1:3) = sum(pressureVect);

tmp1 = ones(length(center(:,1)),1);
tmp2 = tmp1*instcg';
center2cgVec = center-tmp2;

f(4:6)= sum(cross(center2cgVec,pressureVect));
end

== matlab function MPS_device_passive/PTO P3F3/VisuP3F2/Hydrodynamic Body/Morrison Element and ViscousDampingForceCalculation/Morrison Element Variant Subsystem/Morrison Element On/Irregular Wave Morison Force/MorrisonElements/MorisonElementIrregular/MATLAB Function ==
  data: u output; v output; disp input size=[1 3]; waveNumber input; waveFreq input; waveAmp input; randPhase input; time input; rampT input size=[1 1]; waveDir input size=[1 1]; waterDepth input size=[1 1]; g input size=[1 1]; w output; xa output; ya output; za output
function [u,v,w,xa,ya,za] = calc_orbital_vel(disp, waveNumber, waveFreq, waveAmp, randPhase, time, rampT, waveDir, waterDepth, g)
%#codegen

[u,v,w,xa,ya,za] = orbital_velocity(disp, waveNumber, waveFreq, waveAmp, randPhase, time, rampT, waveDir, waterDepth, g);

== matlab function MPS_device_passive/PTO P3F3/VisuP3F2/Hydrodynamic Body/Morrison Element and ViscousDampingForceCalculation/Morrison Element Variant Subsystem/Morrison Element On/Regular Wave Morison Force/MorrisonElements/OrbitalVelocity/MATLAB Function ==
  data: u output; v output; disp input size=[1 3]; waveNumber input size=[1 1]; waveFreq input size=[1 1]; waveAmp input size=[1 1]; randPhase input; time input; rampT input size=[1 1]; waveDir input size=[1 1]; waterDepth input size=[1 1]; g input size=[1 1]; w output; xa output; ya output; za output
function [u,v,w,xa,ya,za] = calc_orbital_vel(disp, waveNumber, waveFreq, waveAmp, randPhase, time, rampT, waveDir, waterDepth, g)
%#codegen

[u,v,w,xa,ya,za] = orbital_velocity(disp, waveNumber, waveFreq, waveAmp, randPhase, time, rampT, waveDir, waterDepth, g);

== matlab function MPS_device_passive/PTO P3F3/VisuP3F2/Hydrodynamic Body/Nonlinear Wave Elevation/Linear or Instantaneous Free Surface/Instantaneous Water Free Surface  /Instantaneous FS ==
  data: x input; center input; f output; cg input; AH input; w input; dw input; k input; typeNum input; t input; rampT input; phaseRand input; waveDir input; dt input; dtFe input
function f  = waveElevation(x,center,cg,AH,w,dw,k,typeNum,t,rampT,phaseRand,waveDir, dt, dtFe)
    % Function to calculate the wave elevation at the ceontroids of triangulated surface
    % NOTE: This function assumes that the STL file is imported with its CG at 0,0,0
    persistent oldElev
    if isempty(oldElev)
        f = calc_elev(x,center,cg,AH,w,dw,k,typeNum,t,rampT,phaseRand, waveDir);
        oldElev = f;
    else
        if mod(t, dtFe) < dt/2
            f = calc_elev(x,center,cg,AH,w,dw,k,typeNum,t,rampT,phaseRand, waveDir);
            oldElev = f;
        else
            f = oldElev;
        end
    end
end

function f = calc_elev(x,center,cg,AH,w,dw,k,typeNum,t,rampT,phaseRand,waveDir)
    % Function to rotate and translate body and call wave elevation function at new locations 
    
    % Compute new tri center coords after cog rotation and translation
    center = rotateXYZ(center,[1 0 0],x(4));
    center = rotateXYZ(center,[0 1 0],x(5));
    center = rotateXYZ(center,[0 0 1],x(6));
    center = offsetXYZ(center,x);
    center = offsetXYZ(center,cg);
    % Calculate the free surface
    f=waveElev(center,AH,w,dw,t,k,rampT,phaseRand,typeNum,waveDir);
end

function verts = offsetXYZ(verts,x)
    % Function to move the position vertices
    verts(:,1) = verts(:,1) + x(1);
    verts(:,2) = verts(:,2) + x(2);
    verts(:,3) = verts(:,3) + x(3);
end

function xn = rotateXYZ(x,ax,t)
	% Function to rotate a point about an arbitrary axis
	% x: 3-component coordinates
	% ax: axis about which to rotate (must be a vector length 1)
	% t: rotation angle
	% xn: new coordinates after rotation
	rotMat = zeros(3);
	rotMat(1,1) = ax(1)*ax(1)*(1-cos(t))    + cos(t);
	rotMat(1,2) = ax(2)*ax(1)*(1-cos(t))    + ax(3)*sin(t);
	rotMat(1,3) = ax(3)*ax(1)*(1-cos(t))    - ax(2)*sin(t);
	rotMat(2,1) = ax(1)*ax(2)*(1-cos(t))    - ax(3)*sin(t);
	rotMat(2,2) = ax(2)*ax(2)*(1-cos(t))    + cos(t);
	rotMat(2,3) = ax(3)*ax(2)*(1-cos(t))    + ax(1)*sin(t);
	rotMat(3,1) = ax(1)*ax(3)*(1-cos(t))    + ax(2)*sin(t);
	rotMat(3,2) = ax(2)*ax(3)*(1-cos(t))    - ax(1)*sin(t);
	rotMat(3,3) = ax(3)*ax(3)*(1-cos(t))    + cos(t);
	xn = x*rotMat;
end

function f=waveElev(center,AH,w,dw,t,k,rampT,phaseRand,typeNum,waveDir)
    % Function to calculate the wave elevation at an array of points
    f = zeros(length(center(:,3)),1);
    cx = center(:,1);
    cy = center(:,2);
    X = cx*cos(waveDir*pi/180) + cy*sin(waveDir*pi/180);
    if typeNum <10
    elseif typeNum <20
        f = AH(1).*cos(k(1).*X-w(1)*t);
    elseif typeNum <30
        tmp=sqrt(AH.*dw);
        tmp1 = ones(1,length(center(:,1)));
        tmp2 = (w.*t+phaseRand)*tmp1;
        tmp3 = cos(k*X'- tmp2);
        f(:,1) = tmp3'*tmp;
    end
    if t<=rampT
        rampF = (1+cos(pi+pi*t/rampT))/2;
        f = f.*rampF;
    end
end

== matlab function MPS_device_passive/PTO P3F3/VisuP3F2/Hydrodynamic Body/Structure/Motion Sensor/Angle ==
  data: Q input; E output
function E  = EulerAngle(Q)
% Euler Angle Type II or Tait-Bryan Angle for sequence 321 or zyx (Nautical or Cardan angles).
% Yaw [-180,180], followed by pitch [-90,90], followed by roll [-180,180]
E = zeros(3,1);
E(1) = atan2((2*(Q(1)*Q(2)+Q(3)*Q(4))),(1-2*(Q(2)^2+Q(3)^2)));
E(2) = asin(2*(Q(1)*Q(3)-Q(4)*Q(2)));
E(3) = atan2((2*(Q(1)*Q(4)+Q(2)*Q(3))),(1-2*(Q(3)^2+Q(4)^2)));

== matlab function MPS_device_passive/PTO P3F3/VisuP3F2/Hydrodynamic Body/Wave Diffraction and Excitation Force Calculation/Linear Wave Excitation Force Variant Subsystem/Irregular Wave Excitation Force/MATLAB Function ==
  data: A input; Fext output; w input; fExtRE input; fExtIM input; phaseRand input; dw input; time input
function Fext = fcn(A,w,fExtRE,fExtIM,phaseRand,dw,time)
%#codegen

persistent A1 B1 B11 C1 D1 D11 E1 E11

A1=bsxfun(@plus,w*time,pi/2);
B1= sin(bsxfun(@plus,A1,phaseRand));
B11 = sin(bsxfun(@plus,w*time,phaseRand));
C1 = sqrt(bsxfun(@times,A,dw));
D1 =bsxfun(@times,fExtRE,C1);
D11 = bsxfun(@times,fExtIM,C1);
E1 = bsxfun(@times,B1,D1);
E11 = bsxfun(@times,B11,D11);

Fext = sum(bsxfun(@minus,E1,E11));

== matlab function MPS_device_passive/PTO P3F3/VisuP3F2/Hydrodynamic Body/Wave Diffraction and Excitation Force Calculation/Nonlinear FK Force Variant Subsystem/With Nonlinear FroudeKrylov Force/Diffraction and Excitation Forces ==
  data: x input; elv input; center input; f output; tnorm input; area input; rho input; g input; cg input; AH input; w input; dw input; wDepth input; deepWaterWave input; k input; typeNum input; t input; phaseRand input; wp output; wpMeanFS output; dt input; dtFe input
function [f, wp, wpMeanFS]  = nonFKForce(x,elv,center,tnorm,area,rho,g,cg,AH,w,dw,wDepth,deepWaterWave,k,typeNum,t,phaseRand, dt, dtFe)
    % Function to calculate wave exitation force and moment on a triangulated surface
    % NOTE: This function assumes that the STL file is imported with its CG at 0,0,0
    
    % Logic to calculate nonFKForce at reduced sample time
    persistent oldForce
    persistent oldWp
    persistent oldWpMeanFs
    
    if isempty(oldForce)
        [f, wp, wpMeanFS] = calc_force(x,elv,center,tnorm,area,rho,g,cg,AH,w,dw,wDepth,deepWaterWave,k,typeNum,t,phaseRand);
        oldForce = f;
        oldWp = wp;
        oldWpMeanFs = wpMeanFS;
    else
        if mod(t, dtFe) < dt/2
            [f, wp, wpMeanFS] = calc_force(x,elv,center,tnorm,area,rho,g,cg,AH,w,dw,wDepth,deepWaterWave,k,typeNum,t,phaseRand);
            oldForce = f;
            oldWp = wp;
            oldWpMeanFs = wpMeanFS;
        else
            f = oldForce;
            wp = oldWp;
            wpMeanFS = oldWpMeanFs;
        end
    end
end

function [f, wp, wpMeanFS]  = calc_force(x,elv,center,tnorm,area,rho,g,cg,AH,w,dw,wDepth,deepWaterWave,k,typeNum,t,phaseRand)
    % Function to apply translation and rotation, and calculate forces.
    
    % Compute new tri coords after cog rotation and translation
    centerMeanFS = offsetXYZ(center,cg);
    avMeanFS     = tnorm .* [area area area];
    
    % Compute new tri coords after cog rotation and translation
    center = rotateXYZ(center,[1 0 0],x(4));
    center = rotateXYZ(center,[0 1 0],x(5));
    center = rotateXYZ(center,[0 0 1],x(6));
    center = offsetXYZ(center,x);
    center = offsetXYZ(center,cg);
    % Compute new normal vectors coords after cog rotation and translation
    tnorm = rotateXYZ(tnorm,[1 0 0],x(4));
    tnorm = rotateXYZ(tnorm,[0 1 0],x(5));
    tnorm = rotateXYZ(tnorm,[0 0 1],x(6));
    
    % Copute area vectors
    av = tnorm .* [area area area];
    
    % Calculate the free surface
    wpMeanFS=pDis(centerMeanFS,       0,AH,w,dw,wDepth,deepWaterWave,t,k,phaseRand,typeNum,rho,g);
    wp      =pDis(center      ,     elv,AH,w,dw,wDepth,deepWaterWave,t,k,phaseRand,typeNum,rho,g);
    
    % Calculate forces
    f_linear   =FK(centerMeanFS,       cg,avMeanFS,wpMeanFS);
    f_nonLinear=FK(center      ,x(1:3)+cg,av      ,wp      ); 
    f = f_nonLinear-f_linear;
end

function verts = offsetXYZ(verts,x)
    % Function to move the position vertices
    verts(:,1) = verts(:,1) + x(1);
    verts(:,2) = verts(:,2) + x(2);
    verts(:,3) = verts(:,3) + x(3);
end

function xn = rotateXYZ(x,ax,t)
	% Function to rotate a point about an arbitrary axis
	% x: 3-componenet coordinates
	% ax: axis about which to rotate (must be a vector length 1)
	% t: rotation angle
	% xn: new coordinates after rotation
	rotMat = zeros(3);
	rotMat(1,1) = ax(1)*ax(1)*(1-cos(t))    + cos(t);
	rotMat(1,2) = ax(2)*ax(1)*(1-cos(t))    + ax(3)*sin(t);
	rotMat(1,3) = ax(3)*ax(1)*(1-cos(t))    - ax(2)*sin(t);
	rotMat(2,1) = ax(1)*ax(2)*(1-cos(t))    - ax(3)*sin(t);
	rotMat(2,2) = ax(2)*ax(2)*(1-cos(t))    + cos(t);
	rotMat(2,3) = ax(3)*ax(2)*(1-cos(t))    + ax(1)*sin(t);
	rotMat(3,1) = ax(1)*ax(3)*(1-cos(t))    + ax(2)*sin(t);
	rotMat(3,2) = ax(2)*ax(3)*(1-cos(t))    - ax(1)*sin(t);
	rotMat(3,3) = ax(3)*ax(3)*(1-cos(t))    + cos(t);
	xn = x*rotMat;
end

function f=pDis(center,elv,AH,w,dw,wDepth,deepWaterWave,t,k,phaseRand,typeNum,rho,g)
    % Function to calculate pressure distribution
    f = zeros(length(center(:,3)),1);
    z=zeros(length(center(:,1)),1);
    if typeNum <10
    elseif typeNum <20
        f = rho.*g.*AH(1).*cos(k(1).*center(:,1)-w(1)*t);
        if deepWaterWave == 0
            z=(center(:,3)-elv).*wDepth./(wDepth+elv);
            f = f.*(cosh(k(1).*(z+wDepth))./cosh(k(1)*wDepth));
        else
            z=(center(:,3)-elv);
            f = f.*exp(k(1).*z);
        end
    elseif typeNum <30
        for i=1:length(AH)
            if deepWaterWave == 0 && wDepth <= 0.5*pi/k(i)
                z=(center(:,3)-elv).*wDepth./(wDepth+elv);
                f_tmp = rho.*g.*sqrt(AH(i)*dw).*cos(k(i).*center(:,1)-w(i)*t-phaseRand(i));
                f = f + f_tmp.*(cosh(k(i).*(z+wDepth))./cosh(k(i).*wDepth));
            else
                z=(center(:,3)-elv);
                f_tmp = rho.*g.*sqrt(AH(i)*dw).*cos(k(i).*center(:,1)-w(i)*t-phaseRand(i));
                f = f + f_tmp.*exp(k(i).*z);
            end
        end
    end
    f(z>0)=0;
end

function f = FK(center,instcg,av,wp)
    % Function to calculate the force and moment about the cog due to Froude-Krylov pressure
    f = zeros(6,1);
    
    % Calculate the hydrostatic pressure at each triangle center
    pressureVect = [wp wp wp].*-av;
    
    % Compute force about cog
    f(1:3) = sum(pressureVect);
    
    % Compute moment about cog
    tmp1 = ones(length(center(:,1)),1);
    tmp2 = tmp1*instcg';
    center2cgVec = center-tmp2;
    
    f(4:6)= sum(cross(center2cgVec,pressureVect));
end

== matlab function MPS_device_passive/PTO P3F3/VisuP3F2/Hydrodynamic Body/Wave Radiation Forces Calculation/SS CI and Constant-Damping-CoeVariant Subsystem/Convolution Integral Calculation/Fluid Memory ==
  data: lenJ input; v input; F_FM output; IRKB input; CTTime input; clockTime input
function F_FM = ConvolutionIntegral(lenJ,v,IRKB,CTTime,clockTime)
% Function to calculate convolution integral
interp_factor = 1;
%define persistent variables
persistent velocity;
persistent oldTime;
persistent oldF_FM;
persistent IRKB_interp;

dt = CTTime(2)-CTTime(1);
len = length(CTTime);
lenJ=length(lenJ);

%update velocity
if isempty(velocity)
    velocity = zeros(lenJ,len);
    oldTime = 0;
    F_FM    = zeros(6,1);
    oldF_FM = zeros(6,1);
    IRKB_reordered = permute(IRKB,[3 1 2]);
    IRKB_interp    = IRKB_reordered(:,1:interp_factor:end, :);
else
    if abs(clockTime-oldTime-dt)<0.00000001
        velocity      = circshift(velocity, 1, 2);
        velocity(:,1) = v(:);
        %integrate       
        time_series = bsxfun(@times, IRKB_interp, velocity);
        F_FM =squeeze(trapz(CTTime,sum(time_series, 1)));
         oldF_FM = F_FM;
         oldTime = clockTime;
    else
        F_FM = oldF_FM;
    end
end

end

== matlab function MPS_device_passive/PTO P3F3/VisuP3F2/Non-Hydro Body/Structure/Motion Sensor/Angle ==
  data: Q input; E output
function E  = EulerAngle(Q)
% Euler Angle Type II or Tait-Bryan Angle for sequence 321 or zyx (Nautical or Cardan angles).
% Yaw [-180,180], followed by pitch [-90,90], followed by roll [-180,180]
E = zeros(3,1);
E(1) = atan2( (2*(Q(1)*Q(2)+Q(3)*Q(4))), (1-2* (Q(2)^2+Q(3)^2) ) );
E(2) = asin( 2* (Q(1)*Q(3) - Q(4)*Q(2)));
E(3) = atan2( (2*(Q(1)*Q(4)+Q(2)*Q(3))), (1-2* (Q(3)^2+Q(4)^2) ) );
